simulink model "HDL_DUC"  (R2024a)
settings: Solver=VariableStepAuto  StartTime=0.0  StopTime=sample_period*512*150  RelTol=1e-3
InitFcn:
  | sample_period=1/400e6;
  | coeffs_scaling;
  | dds=80e6; % ddfs frequency
undefined symbols (not defined in the file or in its folder): S, vsva2197, xcvc1902
libraries: hdlBasic x13, hdlDSPIP x6, dspmlti4 x4, vmcUtilities x1
settings Model: Creator=mmi  LastModifiedBy=robg
settings DebuggingCC: ParameterOverflowMsg=warning  UnconnectedInputMsg=warning  UnconnectedOutputMsg=warning  UnconnectedLineMsg=warning
settings HardwareCC: ProdBitPerPointer=32  ProdBitPerSizeT=32  ProdBitPerPtrDiffT=32  ProdLargestAtomicFloat=None  ProdIntDivRoundTo=Undefined  ProdEndianess=Unspecified  ProdWordSize=32  ProdHWDeviceType=ASIC/FPGA->ASIC/FPGA  TargetBitPerLong=64  TargetBitPerPointer=64  TargetBitPerSizeT=64  TargetBitPerPtrDiffT=64  TargetLongLongMode=on  TargetIntDivRoundTo=Zero  TargetEndianess=LittleEndian  TargetWordSize=64  TargetHWDeviceType=Custom Processor->MATLAB Host Computer  ProdEqTarget=off
settings ModelReferenceCC: EnableRefExpFcnMdlSchedulingChecks=on
settings RTWCC: GPUComputeCapability=3.5  DLArmComputeVersion=19.05

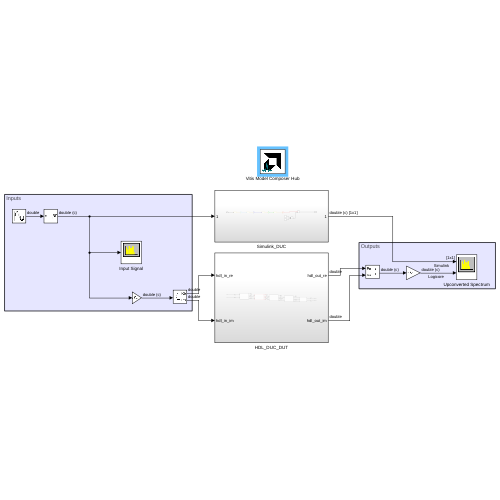
[thumbnail: Simulink's stored preview of the top-level diagram]
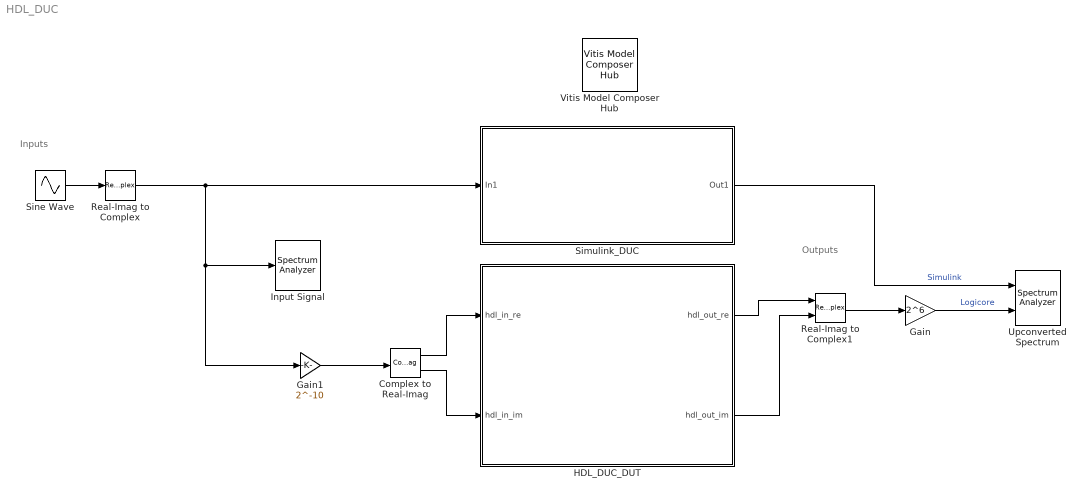
== system HDL_DUC ==
  note: Outputs
  note: Inputs
  Complex to Real-Imag : ComplexToRealImag
  Gain : Gain  Gain=2^6
  Gain1 : Gain  Gain=2^-10  RndMeth=Convergent  OutDataTypeStr=Inherit: Same as input
  HDL_DUC_DUT : Subsystem
  Input Signal : SpectrumAnalyzer  WindowPosition=[880.000000,430.000000,800.000000,500.000000,]  Visible=on  ScopeFrameLocation=window  YLimits=[0.3303,93.2493]
  Real-Imag to Complex : RealImagToComplex  Input=Real
  Real-Imag to Complex1 : RealImagToComplex
  Simulink_DUC : Subsystem
  Sine Wave : Sin  Amplitude=1000  Frequency=2*pi*1e6  SampleTime=16*sample_period
  Upconverted Spectrum : SpectrumAnalyzer  NumInputPorts=2  WindowPosition=[144.000000,133.000000,820.000000,457.000000,]  Visible=on  ScopeFrameLocation=window  SampleRate=400000000  AxesScaling=Manual  Span=400000000  StartFrequency=-200000000  StopFrequency=200000000  AveragingMethod=Exponential  YLimits=[53.99482462462336,141.04233735662578]  ShowLegend=on  AllowFFTLengthLessThanSamplesPerUpdate=on
  Vitis Model Composer Hub : vmcUtilities/Vitis Model Composer Hub  Tag=genX  CodeGeneration=off  SubsystemName=HDL_DUC_DUT  CompilationType=HDLCompilation  SubsystemType=HDLNode  ExportTypeV2=IP Catalog  StartColumn=1  NumberOfColumns=1  TargetDirectory=./netlist  exportDesign=off  analyzeDesign=on  validateDesignOnHw=off  ExportType=AI Engines  IpVendor=xilinx.com  IpLibrary=hls  IpVersion=1.0  IpHWLanguage=Verilog  AieCompilerOptions={}  AieSimulatorOptions={}  CreateTestbench=on  TestbenchStackSize=10  RunRtlSim=off  RunCSim=off  RunAieSim=on  AieSimTimeout=50000  RunAieSimProfiling=off  LaunchVitisAnalyzer=on  PlotOutput=off  RunX86Sim=off  X86SimTimeout=10  GenHwImage=off  GenLibadfXo=off  GenHwValidationCode=off  PlatformType=Not Specified  HwSystemType=Baremetal  HwValidationTarget=hw  ProjDevice=Versal VCK190 Evaluation Platform with New SD Level Shifter (xcvc1902-vsva2197-2MP-e-S)  ProjDevicePart=xcvc1902-vsva2197-2MP-e-S  AIEType=AIE  SamplePeriod=-1  ClockFrequency=200  DataPathParallelism=1  xilinxfamily=versalaicore  part=xcvc1902  speed=-2MP-e-S  package=vsva2197  directory=./netlist/ip/HDL_DUC_DUT/src  testbench=on  incr_netlist=off  synthesis_tool=Vivado  clock_wrapper=Clock Enables  dbl_ovrd=According to Block Masks  dcm_input_clock_period=10  sysclk_period=1.25  simulink_period=sample_period  eval_field=0  IPInfoJsonString="{\"DUTSubsystemName\":\"HDL_DUC_DUT\",\"HDLSubsystem\":{\"SubsystemName\":\"HDL_DUC_DUT\",\"IPName\":\"HDL_DUC\",\"IPLibrary\":\"VMC\",\"IPVendor\":\"User Company\",\"IPVersion\":\"1.0\",\"TargetDirectory\":\"./netlist\",\"SubsystemDir\":\"./netlist/ip/HDL_DUC_DUT\",\"FreqHz\":\"800000000\"},\"SubsystemTag\":\"HDLNode\"}"  LogFileName=/group/xcoswmktg2/robg/git/vmc_examples/github-fork/Examples/HDL/RFSoC/HDL_DUC/netlist/model_composer.log  NThreads=4  IPConfigFile=/tmp/vmctmp-robg/247401/ipconfig.json
  wires:
  Real-Imag to Complex/1 -> Input Signal/1, Gain1/1, Simulink_DUC/1(In1)
  Complex to Real-Imag/1 -> HDL_DUC_DUT/1(hdl_in_re)
  Complex to Real-Imag/2 -> HDL_DUC_DUT/2(hdl_in_im)
  Sine Wave/1 -> Real-Imag to Complex/1
  Gain1/1 -> Complex to Real-Imag/1
  HDL_DUC_DUT/1(hdl_out_re) -> Real-Imag to Complex1/1
  Simulink_DUC/1(Out1) -> Upconverted Spectrum/1  "Simulink"
  Real-Imag to Complex1/1 -> Gain/1
  HDL_DUC_DUT/2(hdl_out_im) -> Real-Imag to Complex1/2
  Gain/1 -> Upconverted Spectrum/2  "Logicore"

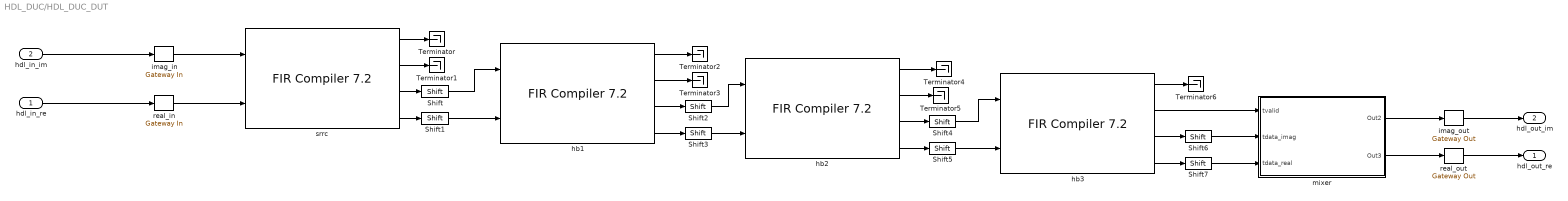
== system HDL_DUC/HDL_DUC_DUT ==
  hdl_in_re : Inport
  hdl_in_im : Inport  Port=2
  Shift{,1..7} (8 alike) : hdlBasic/Shift  shift_dir=Left  shift_bits=1  en=off  latency=0  precision=Full  arith_type="Signed  (2's comp)"  n_bits=16  bin_pt=14  quantization=Truncate  overflow=Wrap  XmcBlockStatus=1  maskContainerNames=group2  block_type=shift  block_config=sysgen:Shift_config
  Terminator{,1..6} (7 alike) : Terminator
  hb1 : hdlDSPIP/FIR Compiler 7.2   coefficientvector=hb1_coeff  coefficient_sets=1  coefficient_reload=off  filter_type=Interpolation  rate_change_type=Integer  interpolation_rate=2  decimation_rate=1  zero_pack_factor=1  channel_sequence=Basic  number_channels=1  pattern_list='P4-0,P4-1,P4-2,P4-3,P4-4'  number_paths=2  ratespecification=Maximum_Possible  sampleperiod=16  hardwareoversamplingrate=1  coefficient_sign=Signed  quantization=Maximize_Dynamic_Range  coefficient_width=17  bestprecision=on  coefficient_fractional_bits=0  coefficient_structure=Inferred  output_rounding_mode=Truncate_LSBs  output_width=17  filter_architecture=Systolic_Multiply_Accumulate  optimization_goal=Area  optimization_list='None'  data_buffer_type=Automatic  coefficient_buffer_type=Automatic  input_buffer_type=Automatic  output_buffer_type=Automatic  preference_for_other_storage=Automatic  multi_column_support=Automatic  columnconfig='3'  inter_column_pipe_length=4  data_has_tlast=Not_Required  m_data_has_tready=off  s_data_has_fifo=off  s_data_has_tuser=Not_Required  m_data_has_tuser=Not_Required  s_config_sync_mode=On_Vector  s_config_method=Single  num_reload_slots=1  has_aclken=off  has_aresetn=off  reset_data_vector=on  trim_axipin_name=on  simulation_type=hybrid_sim  simulation_model=sysgen:xfirv7_2_cmodel  data_path_portlist={ 's_axis_data_tdata', 'm_axis_data_tdata' }  passband_min=0.0  passband_max=0.5  stopband_min=0.5  stopband_max=1.0  filter_selection=1  gui_behaviour='Sysgen_GUI'  data_sign=Signed  data_width=16  data_fractional_bits=0  data_tuser_width=1  wrapper_available=true  ip_wrap_arbitrary_binary_point=true  ip_name=FIR Compiler  ip_version=7.2  dsptool_ready=true  ipcore_usecache=true  ipcore_useipmodelcache=true  port_translation_map={ 'aclken' => 'en', 'aresetn' => 'rst' }  run_core_at_system_period=true  ipcore_xco_need_fpga_part=true  ipcore_fpga_part=[]  XmcBlockStatus=1  maskContainerNames=tabcontainer1  block_type=fir_compiler_v7_2  block_config=sysgen:rodinimport_config  block_width=820  block_height=600
  hb2 : hdlDSPIP/FIR Compiler 7.2   coefficientvector=hb2_coeff  coefficient_sets=1  coefficient_reload=off  filter_type=Interpolation  rate_change_type=Integer  interpolation_rate=2  decimation_rate=1  zero_pack_factor=1  channel_sequence=Basic  number_channels=1  pattern_list='P4-0,P4-1,P4-2,P4-3,P4-4'  number_paths=2  ratespecification=Maximum_Possible  sampleperiod=16  hardwareoversamplingrate=1  coefficient_sign=Signed  quantization=Maximize_Dynamic_Range  coefficient_width=17  bestprecision=on  coefficient_fractional_bits=17  coefficient_structure=Inferred  output_rounding_mode=Truncate_LSBs  output_width=17  filter_architecture=Systolic_Multiply_Accumulate  optimization_goal=Area  optimization_list='None'  data_buffer_type=Automatic  coefficient_buffer_type=Automatic  input_buffer_type=Automatic  output_buffer_type=Automatic  preference_for_other_storage=Automatic  multi_column_support=Automatic  columnconfig='2'  inter_column_pipe_length=4  data_has_tlast=Not_Required  m_data_has_tready=off  s_data_has_fifo=off  s_data_has_tuser=Not_Required  m_data_has_tuser=Not_Required  s_config_sync_mode=On_Vector  s_config_method=Single  num_reload_slots=1  has_aclken=off  has_aresetn=off  reset_data_vector=on  trim_axipin_name=on  simulation_type=hybrid_sim  simulation_model=sysgen:xfirv7_2_cmodel  data_path_portlist={ 's_axis_data_tdata', 'm_axis_data_tdata' }  passband_min=0.0  passband_max=0.5  stopband_min=0.5  stopband_max=1.0  filter_selection=1  gui_behaviour='Sysgen_GUI'  data_sign=Signed  data_width=16  data_fractional_bits=0  data_tuser_width=1  wrapper_available=true  ip_wrap_arbitrary_binary_point=true  ip_name=FIR Compiler  ip_version=7.2  dsptool_ready=true  ipcore_usecache=true  ipcore_useipmodelcache=true  port_translation_map={ 'aclken' => 'en', 'aresetn' => 'rst' }  run_core_at_system_period=true  ipcore_xco_need_fpga_part=true  ipcore_fpga_part=[]  XmcBlockStatus=1  maskContainerNames=tabcontainer1  block_type=fir_compiler_v7_2  block_config=sysgen:rodinimport_config  block_width=820  block_height=600
  hb3 : hdlDSPIP/FIR Compiler 7.2   coefficientvector=hb3_coeff  coefficient_sets=1  coefficient_reload=off  filter_type=Interpolation  rate_change_type=Integer  interpolation_rate=2  decimation_rate=1  zero_pack_factor=1  channel_sequence=Basic  number_channels=1  pattern_list='P4-0,P4-1,P4-2,P4-3,P4-4'  number_paths=2  ratespecification=Maximum_Possible  sampleperiod=16  hardwareoversamplingrate=1  coefficient_sign=Signed  quantization=Maximize_Dynamic_Range  coefficient_width=17  bestprecision=on  coefficient_fractional_bits=17  coefficient_structure=Inferred  output_rounding_mode=Truncate_LSBs  output_width=17  filter_architecture=Systolic_Multiply_Accumulate  optimization_goal=Area  optimization_list='None'  data_buffer_type=Automatic  coefficient_buffer_type=Automatic  input_buffer_type=Automatic  output_buffer_type=Automatic  preference_for_other_storage=Automatic  multi_column_support=Automatic  columnconfig='1'  inter_column_pipe_length=4  data_has_tlast=Not_Required  m_data_has_tready=off  s_data_has_fifo=off  s_data_has_tuser=Not_Required  m_data_has_tuser=Not_Required  s_config_sync_mode=On_Vector  s_config_method=Single  num_reload_slots=1  has_aclken=off  has_aresetn=off  reset_data_vector=on  trim_axipin_name=on  simulation_type=hybrid_sim  simulation_model=sysgen:xfirv7_2_cmodel  data_path_portlist={ 's_axis_data_tdata', 'm_axis_data_tdata' }  passband_min=0.0  passband_max=0.5  stopband_min=0.5  stopband_max=1.0  filter_selection=1  gui_behaviour='Sysgen_GUI'  data_sign=Signed  data_width=16  data_fractional_bits=0  data_tuser_width=1  wrapper_available=true  ip_wrap_arbitrary_binary_point=true  ip_name=FIR Compiler  ip_version=7.2  dsptool_ready=true  ipcore_usecache=true  ipcore_useipmodelcache=true  port_translation_map={ 'aclken' => 'en', 'aresetn' => 'rst' }  run_core_at_system_period=true  ipcore_xco_need_fpga_part=true  ipcore_fpga_part=[]  XmcBlockStatus=1  maskContainerNames=tabcontainer1  block_type=fir_compiler_v7_2  block_config=sysgen:rodinimport_config  block_width=820  block_height=600
  imag_in : hdlBasic/Gateway In  gui_display_data_type=Fixed-point  arith_type=Signed (2's comp)  n_bits=17  bin_pt=14  preci_type=Single  exp_width=8  frac_width=24  rows=1  columns=1  quantization=Truncate  overflow=Wrap  period=sample_period*16  UseAsADC=off  ADCChannel='1'  interface=None  automatic_assignment=on  address_offset=hex2dec('00')  intf_name=''  intf_description=''  default_value=0  timing_constraint=None  locs_specified=off  LOCs={}  io_standard={}  inherit_from_input=off  hdl_port=on  XmcBlockStatus=1  maskContainerNames=group4  block_type=gatewayin  block_config=sysgen:gateway_in_config  block_width_w=590  block_height_w=620  block_width=640  block_height=850
  imag_out : hdlBasic/Gateway Out  inherit_from_input=off  hdl_port=on  rows=1  columns=1  UseAsDAC=off  DACChannel='1'  interface=None  automatic_assignment=on  address_offset=hex2dec('00')  intf_name=''  intf_description=''  timing_constraint=None  locs_specified=off  LOCs={}  io_standard={}  XmcBlockStatus=1  maskContainerNames=group4  block_type=gatewayout  block_config=sysgen:gateway_out_config  block_width_w=590  block_height_w=620  block_width=620  block_height=750
  mixer : Subsystem
  real_in : hdlBasic/Gateway In  gui_display_data_type=Fixed-point  arith_type=Signed (2's comp)  n_bits=17  bin_pt=14  preci_type=Single  exp_width=8  frac_width=24  rows=1  columns=1  quantization=Truncate  overflow=Wrap  period=sample_period*16  UseAsADC=off  ADCChannel='1'  interface=None  automatic_assignment=on  address_offset=hex2dec('00')  intf_name=''  intf_description=''  default_value=0  timing_constraint=None  locs_specified=off  LOCs={}  io_standard={}  inherit_from_input=off  hdl_port=on  XmcBlockStatus=1  maskContainerNames=group4  block_type=gatewayin  block_config=sysgen:gateway_in_config  block_width_w=590  block_height_w=620  block_width=640  block_height=850
  real_out : hdlBasic/Gateway Out  inherit_from_input=off  hdl_port=on  rows=1  columns=1  UseAsDAC=off  DACChannel='1'  interface=None  automatic_assignment=on  address_offset=hex2dec('00')  intf_name=''  intf_description=''  timing_constraint=None  locs_specified=off  LOCs={}  io_standard={}  XmcBlockStatus=1  maskContainerNames=group4  block_type=gatewayout  block_config=sysgen:gateway_out_config  block_width_w=590  block_height_w=620  block_width=620  block_height=750
  srrc : hdlDSPIP/FIR Compiler 7.2   coefficientvector=srrc_coeff  coefficient_sets=1  coefficient_reload=off  filter_type=Interpolation  rate_change_type=Integer  interpolation_rate=2  decimation_rate=1  zero_pack_factor=1  channel_sequence=Basic  number_channels=1  pattern_list='P4-0,P4-1,P4-2,P4-3,P4-4'  number_paths=2  ratespecification=Maximum_Possible  sampleperiod=1  hardwareoversamplingrate=1  coefficient_sign=Signed  quantization=Maximize_Dynamic_Range  coefficient_width=17  bestprecision=on  coefficient_fractional_bits=0  coefficient_structure=Inferred  output_rounding_mode=Truncate_LSBs  output_width=17  filter_architecture=Systolic_Multiply_Accumulate  optimization_goal=Area  optimization_list='None'  data_buffer_type=Automatic  coefficient_buffer_type=Automatic  input_buffer_type=Automatic  output_buffer_type=Automatic  preference_for_other_storage=Automatic  multi_column_support=Automatic  columnconfig='33'  inter_column_pipe_length=4  data_has_tlast=Not_Required  m_data_has_tready=off  s_data_has_fifo=off  s_data_has_tuser=Not_Required  m_data_has_tuser=Not_Required  s_config_sync_mode=On_Vector  s_config_method=Single  num_reload_slots=1  has_aclken=off  has_aresetn=off  reset_data_vector=on  trim_axipin_name=on  simulation_type=hybrid_sim  simulation_model=sysgen:xfirv7_2_cmodel  data_path_portlist={ 's_axis_data_tdata', 'm_axis_data_tdata' }  passband_min=0.0  passband_max=0.5  stopband_min=0.5  stopband_max=1.0  filter_selection=1  gui_behaviour='Sysgen_GUI'  data_sign=Signed  data_width=16  data_fractional_bits=0  data_tuser_width=1  wrapper_available=true  ip_wrap_arbitrary_binary_point=true  ip_name=FIR Compiler  ip_version=7.2  dsptool_ready=true  ipcore_usecache=true  ipcore_useipmodelcache=true  port_translation_map={ 'aclken' => 'en', 'aresetn' => 'rst' }  run_core_at_system_period=true  ipcore_xco_need_fpga_part=true  ipcore_fpga_part=[]  XmcBlockStatus=1  maskContainerNames=tabcontainer1  block_type=fir_compiler_v7_2  block_config=sysgen:rodinimport_config  block_width=820  block_height=600
  hdl_out_re : Outport
  hdl_out_im : Outport  Port=2
  wires:
  hb2/2 -> Terminator5/1
  Shift/1 -> hb1/1
  Shift3/1 -> hb2/2
  srrc/2 -> Terminator1/1
  srrc/3 -> Shift/1
  real_out/1 -> hdl_out_re/1
  Shift5/1 -> hb3/2
  hb3/1 -> Terminator6/1
  srrc/1 -> Terminator/1
  hb1/3 -> Shift2/1
  srrc/4 -> Shift1/1
  hdl_in_re/1 -> real_in/1
  hb2/3 -> Shift4/1
  hb3/4 -> Shift7/1
  imag_out/1 -> hdl_out_im/1
  hb2/1 -> Terminator4/1
  hdl_in_im/1 -> imag_in/1
  hb1/1 -> Terminator2/1
  hb1/4 -> Shift3/1
  hb1/2 -> Terminator3/1
  real_in/1 -> srrc/2
  hb3/3 -> Shift6/1
  Shift1/1 -> hb1/2
  imag_in/1 -> srrc/1
  Shift2/1 -> hb2/1
  Shift4/1 -> hb3/1
  hb2/4 -> Shift5/1
  mixer/1(Out2) -> imag_out/1
  mixer/2(Out3) -> real_out/1
  hb3/2 -> mixer/1(tvalid)
  Shift6/1 -> mixer/2(tdata_imag)
  Shift7/1 -> mixer/3(tdata_real)

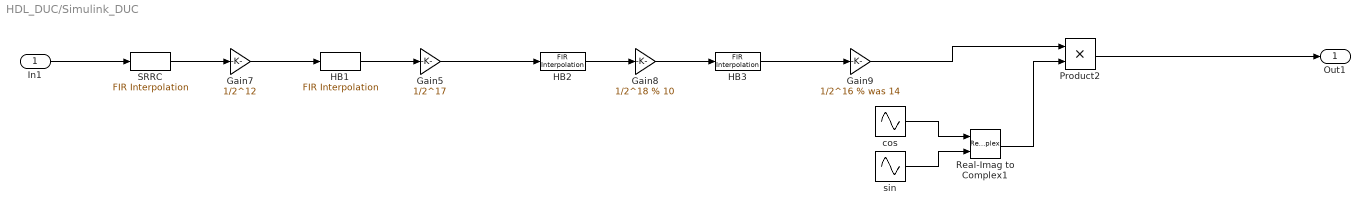
== system HDL_DUC/Simulink_DUC ==
  In1 : Inport
  Gain5 : Gain  Gain=1/2^17  OutDataTypeStr=fixdt(1,32,0)  RndMeth=Convergent
  Gain7 : Gain  Gain=1/2^12  OutDataTypeStr=fixdt(1,32,0)  RndMeth=Convergent
  Gain8 : Gain  Gain=1/2^18 % 10  OutDataTypeStr=fixdt(1,32,0)  RndMeth=Convergent
  Gain9 : Gain  Gain=1/2^16 % was 14  OutDataTypeStr=fixdt(1,32,0)  RndMeth=Convergent
  HB1 : dspmlti4/FIR Interpolation  FilterSource=Dialog parameters  PrivateCoeffs=0  h=hb1_coeff  L=2  FilterObject=FINTERP  framing=Allow multirate processing  outputBufInitCond=0  roundingMode=Floor  overflowMode=off  firstCoeffMode=Specify word length  firstCoeffWordLength=18  firstCoeffFracLength=15  firstCoeffDataTypeStr=fixdt(1,18)  firstCoeffMin=[]  firstCoeffMax=[]  firstCoeffLastDataTypeStr=fixdt(1,18)  outputDataTypeStr=Inherit: Same as accumulator  outputMin=[]  outputMax=[]  outputLastDataTypeStr=Inherit: Same as accumulator
  HB2 : dspmlti4/FIR Interpolation  FilterSource=Dialog parameters  PrivateCoeffs=0  h=hb2_coeff  L=2  FilterObject=FINTERP  framing=Allow multirate processing  outputBufInitCond=0  roundingMode=Floor  overflowMode=off  firstCoeffMode=Specify word length  firstCoeffWordLength=18  firstCoeffFracLength=0  firstCoeffDataTypeStr=fixdt(1,18)  firstCoeffMin=[]  firstCoeffMax=[]  firstCoeffLastDataTypeStr=fixdt(1,18)  outputDataTypeStr=Inherit: Same as accumulator  outputMin=[]  outputMax=[]  outputLastDataTypeStr=Inherit: Same as accumulator
  HB3 : dspmlti4/FIR Interpolation  FilterSource=Dialog parameters  PrivateCoeffs=0  h=hb3_coeff  L=2  FilterObject=FINTERP  framing=Allow multirate processing  outputBufInitCond=0  roundingMode=Floor  overflowMode=off  firstCoeffMode=Specify word length  firstCoeffWordLength=18  firstCoeffFracLength=0  firstCoeffDataTypeStr=fixdt(1,18)  firstCoeffMin=[]  firstCoeffMax=[]  firstCoeffLastDataTypeStr=fixdt(1,18)  outputDataTypeStr=Inherit: Same as accumulator  outputMin=[]  outputMax=[]  outputLastDataTypeStr=Inherit: Same as accumulator
  Product2 : Product
  Real-Imag to Complex1 : RealImagToComplex
  SRRC : dspmlti4/FIR Interpolation  FilterSource=Dialog parameters  PrivateCoeffs=0  h=srrc_coeff  L=2  FilterObject=FINTERP  framing=Allow multirate processing  outputBufInitCond=0  roundingMode=Floor  overflowMode=off  firstCoeffMode=Specify word length  firstCoeffWordLength=18  firstCoeffFracLength=15  firstCoeffDataTypeStr=fixdt(1,18)  firstCoeffMin=[]  firstCoeffMax=[]  firstCoeffLastDataTypeStr=fixdt(1,18)  outputDataTypeStr=Inherit: Same as accumulator  outputMin=[]  outputMax=[]  outputLastDataTypeStr=Inherit: Same as accumulator
  cos : Sin  Frequency=dds*2*pi  Phase=pi/2  SampleTime=sample_period  VectorParams1D=off
  sin : Sin  Frequency=dds*2*pi  SampleTime=sample_period  VectorParams1D=off
  Out1 : Outport
  wires:
  SRRC/1 -> Gain7/1
  cos/1 -> Real-Imag to Complex1/1
  HB1/1 -> Gain5/1
  Real-Imag to Complex1/1 -> Product2/2
  Gain5/1 -> HB2/1
  Gain9/1 -> Product2/1
  Gain8/1 -> HB3/1
  HB2/1 -> Gain8/1
  HB3/1 -> Gain9/1
  Product2/1 -> Out1/1
  Gain7/1 -> HB1/1
  sin/1 -> Real-Imag to Complex1/2
  In1/1 -> SRRC/1

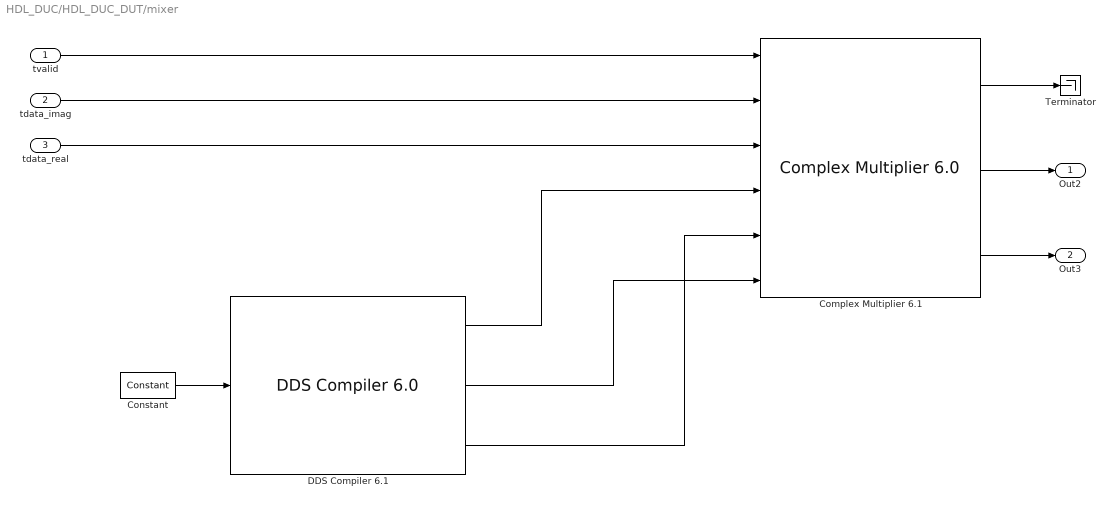
== system HDL_DUC/HDL_DUC_DUT/mixer ==
  tvalid : Inport
  tdata_imag : Inport  Port=2
  tdata_real : Inport  Port=3
  Complex Multiplier 6.1 : hdlDSPIP/Complex Multiplier 6.0   hasatlast=off  hasatuser=off  atuserwidth=1  hasbtlast=off  hasbtuser=off  btuserwidth=1  multtype=Use_Mults  optimizegoal=Performance  flowcontrol=NonBlocking  outputwidth=33  roundmode=Truncate  hasctrltlast=off  hasctrltuser=off  ctrltuserwidth=1  outtlastbehv=Null  latencyconfig=Automatic  minimumlatency=20  aclken=off  aresetn=off  trim_axipin_name=on  simulation_type=hybrid_sim  simulation_model=sysgen:cmpy_v6_0  data_path_portlist={ 's_axis_a_tdata_real', 's_axis_a_tdata_imag', 's_axis_b_tdata_real', 's_axis_b_tdata_imag', 's_axis_ctrl_tdata_rounding_bit', 'm_axis_dout_tdata_real', 'm_axis_dout_tdata_imag' }  aportwidth=63  bportwidth=63  ip_name=Complex Multiplier  ip_version=6.0  dsptool_ready=true  ipcore_usecache=true  ipcore_useipmodelcache=true  ipcore_verbose=false  ipcore_latency_parameter='minimumlatency'  wrapper_available=true  port_translation_map={ 'aclken' => 'en', 'aresetn' => 'rst'}  XmcBlockStatus=1  maskContainerNames=tabcontainer1  block_type=cmpy_v6_0  block_config=sysgen:rodinimport_config
  Constant : hdlBasic/Constant  const=1  gui_display_data_type=Boolean  arith_type=Boolean  n_bits=16  bin_pt=14  preci_type=Single  exp_width=8  frac_width=24  explicit_period=off  period=1  XmcBlockStatus=1  maskContainerNames=tabcontainer1  block_type=constant  block_config=sysgen:Constant_config
  DDS Compiler 6.1 : hdlDSPIP/DDS Compiler 6.0   partspresent=Phase_Generator_and_SIN_COS_LUT  dds_clock_rate=(1/sample_period)/1e6  channels=1  mode_of_operation=Standard  output_type=Integer  modulus=9  parameter_entry=System_Parameters  spurious_free_dynamic_range=85  frequency_resolution=0.07  noise_shaping=Phase_Dithering  phase_width=33  output_width=15  output_selection=Sine_and_Cosine  negative_sine=on  negative_cosine=off  amplitude_mode=Full_Range  memory_type=Auto  optimization_goal=Speed  dsp48_use=Minimal  resync=off  latency_configuration=Auto  latency=1  has_phase_out=off  has_aclken=off  has_aresetn=off  explicit_period=off  period=1  data_has_tlast=Not_Required  has_tready=on  s_phase_has_tuser=Not_Required  m_data_has_tuser=Not_Required  m_phase_has_tuser=Not_Required  s_phase_tuser_width=1  output_form=Twos_Complement  s_config_sync_mode=On_Vector  phase_increment=Fixed  output_frequency1=dds/1e6  output_frequency2=0  output_frequency3=0  output_frequency4=0  output_frequency5=0  output_frequency6=0  output_frequency7=0  output_frequency8=0  output_frequency9=0  output_frequency10=0  output_frequency11=0  output_frequency12=0  output_frequency13=0  output_frequency14=0  output_frequency15=0  output_frequency16=0  pinc1='0'  pinc2='0'  pinc3='0'  pinc4='0'  pinc5='0'  pinc6='0'  pinc7='0'  pinc8='0'  pinc9='0'  pinc10='0'  pinc11='0'  pinc12='0'  pinc13='0'  pinc14='0'  pinc15='0'  pinc16='0'  phase_offset=None  phase_offset_angles1=0  phase_offset_angles2=0  phase_offset_angles3=0  phase_offset_angles4=0  phase_offset_angles5=0  phase_offset_angles6=0  phase_offset_angles7=0  phase_offset_angles8=0  phase_offset_angles9=0  phase_offset_angles10=0  phase_offset_angles11=0  phase_offset_angles12=0  phase_offset_angles13=0  phase_offset_angles14=0  phase_offset_angles15=0  phase_offset_angles16=0  poff1='0'  poff2='0'  poff3='0'  poff4='0'  poff5='0'  poff6='0'  poff7='0'  poff8='0'  poff9='0'  poff10='0'  poff11='0'  poff12='0'  poff13='0'  poff14='0'  poff15='0'  poff16='0'  trim_axipin_name=on  simulation_type=hybrid_sim  simulation_model=sysgen:xddsv6_0_cmodel  data_path_portlist={ 's_axis_config_tdata_poff', 's_axis_config_tdata_chan0_poff', 's_axis_config_tdata_pinc', 's_axis_config_tdata_chan0_pinc', 's_axis_phase_tdata_resync', 's_axis_phase_tdata_chan0_resync', 's_axis_phase_tdata_poff', 's_axis_phase_tdata_chan0_poff', 's_axis_phase_tdata_pinc', 's_axis_phase_tdata_chan0_pinc', 's_axis_phase_tdata_phase_in', 'm_axis_data_tdata_sine', 'm_axis_data_tdata_chan0_sine', 'm_axis_data_tdata_cosine', 'm_axis_data_tdata_chan0_cosine', 'm_axis_phase_tdata_phase_out', 'm_axis_phase_tdata_chan0_phase_out'}  por_mode=false  gui_behaviour=Sysgen  ip_name=DDS Compiler  ip_version=6.0  dsptool_ready=true  wrapper_available=true  port_translation_map={ 'aclken' => 'en', 'aresetn' => 'rst' }  ipcore_usecache=true  ipcore_useipmodelcache=true  ipcore_xco_need_fpga_part=true  ipcore_fpga_part=[]  ipcore_verbose=false  XmcBlockStatus=1  maskContainerNames=tabcontainer1  block_type=dds_compiler_v6_0  block_config=sysgen:rodinimport_config  block_width=760
  Terminator : Terminator
  Out2 : Outport
  Out3 : Outport  Port=2
  wires:
  DDS Compiler 6.1/1 -> Complex Multiplier 6.1/4
  Constant/1 -> DDS Compiler 6.1/1
  Complex Multiplier 6.1/3 -> Out3/1
  DDS Compiler 6.1/2 -> Complex Multiplier 6.1/6
  Complex Multiplier 6.1/1 -> Terminator/1
  DDS Compiler 6.1/3 -> Complex Multiplier 6.1/5
  tvalid/1 -> Complex Multiplier 6.1/1
  Complex Multiplier 6.1/2 -> Out2/1
  tdata_imag/1 -> Complex Multiplier 6.1/2
  tdata_real/1 -> Complex Multiplier 6.1/3
